simulink model "Pendulum"  (R2020b)
settings: Solver=VariableStepAuto  StartTime=0.0  StopTime=20  RelTol=1e-3
values from neighbouring files (symbols this model uses):
  A = [0, 0, 0; 0, 0 , 1; 0, 3*param.g/4/param.l, 0]    [InitPendulumController.m]
  B = [1; 0; 3/4/param.l]    [InitPendulumController.m]
  C = [1, 0, 0; 0, 0, 1]    [InitPendulumController.m]
  L_nom = place(A',C',p_nom)'    [InitPendulumController.m]
  ricatti_controller = lqr(A,B,Q,S)    [InitPendulumController.m]
  T_end = 1.5    [InitPendulumController.m]
  x = double(x1(order))    [InitPendulumController.m]    (also in Visualization.m = -L*sin(phi(idx)))
undefined symbols (not defined in the file or in its folder): ddwandler, DiscIntNeverNeededParam, param, veloctiycontroller
libraries: simulink x5
settings Model: Creator=Rolle  LastModifiedBy=klaus
settings DataIOCC: ReturnWorkspaceOutputs=off
settings DebuggingCC: ArithmeticOperatorsInVariantConditions=warning
settings SFSimCC: SimUseLocalCustomCode=off  CustomCodeUndefinedFunction=UseInterfaceOnly
settings RTWCC: RTWUseLocalCustomCode=off
settings CodeAppCC: StateflowObjectComments=on

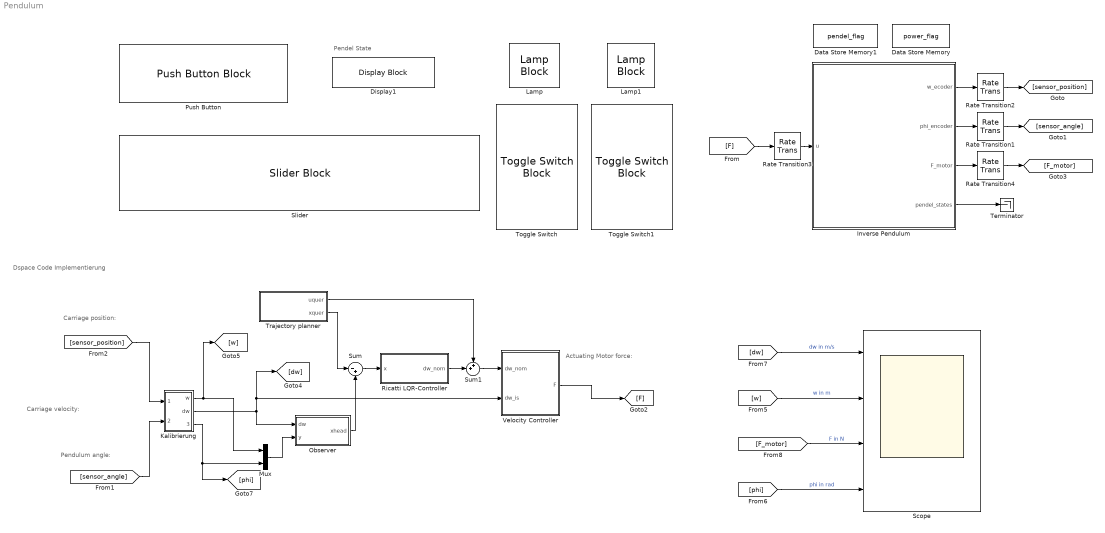
== system Pendulum ==
  note: Carriage position:
  note: Pendel State
  note: Dspace Code Implementierung
  note: Carriage velocity:
  note: Pendulum angle:
  note: Actuating Motor force:
  Data Store Memory : DataStoreMemory  DataStoreName=power_flag  ReadBeforeWriteMsg=warning  WriteAfterWriteMsg=warning  WriteAfterReadMsg=warning  ShowAdditionalParam=off  OutDataTypeStr=boolean
  Data Store Memory1 : DataStoreMemory  DataStoreName=pendel_flag  ReadBeforeWriteMsg=warning  WriteAfterWriteMsg=warning  WriteAfterReadMsg=warning  ShowAdditionalParam=off  OutDataTypeStr=boolean
  Display1 : DisplayBlock  LabelPosition=Hide
  Inverse Pendulum : Subsystem  mask(Inverses Pendel){wagen_flg=off}
      mask prompts: wagen_flg "Aufbau ohne Pendelaufsatz"
      mask help:
      | Schema des stehen Pendels: siehe Skript Abbildung 2.1
      |
      | Kraft ... F
      | Wagenbosition ... w
      | Pendelwinkel ... phi
  Kalibrierung : Subsystem
  Lamp : LampBlock  LabelPosition=Hide
  Lamp1 : LampBlock  LabelPosition=Hide
  Mux : Mux  Inputs=2
  Observer : Subsystem
  Push Button : PushButtonBlock  ButtonText=Disturbe
  Rate Transition1 : RateTransition  OutPortSampleTime=ctr.Ts2
  Rate Transition2 : RateTransition  OutPortSampleTime=ctr.Ts2
  Rate Transition3 : RateTransition
  Rate Transition4 : RateTransition  OutPortSampleTime=ctr.Ts2
  Ricatti LQR-Controller : Subsystem
  Scope : Scope  NumInputPorts=4
  Slider : SliderBlock  ScaleMin=-10  ScaleMax=10
  Sum : Sum  Inputs=|-+
  Sum1 : Sum  Inputs=++|
  Terminator : Terminator
  Toggle Switch : ToggleSwitchBlock
      settings: Values={{'Off', 'On'}, [0 1]}
  Toggle Switch1 : ToggleSwitchBlock
      settings: Values={{'Off', 'On'}, [0 1]}
  Trajectory planner : Subsystem
  Velocity Controller : Subsystem
  wires:
  Inverse Pendulum/2(phi_encoder) -> Rate Transition1/1
  Rate Transition3/1 -> Inverse Pendulum/1(u)
  Inverse Pendulum/1(w_ecoder) -> Rate Transition2/1
  Rate Transition2/1 -> [sensor_position]
  Rate Transition1/1 -> [sensor_angle]
  [F] -> Rate Transition3/1
  Inverse Pendulum/3(F_motor) -> Rate Transition4/1
  Rate Transition4/1 -> [F_motor]
  Inverse Pendulum/4(pendel_states) -> Terminator/1
  Velocity Controller/1(F) -> [F]
  [dw] -> Scope/1  "dw in m/s"
  [w] -> Scope/2  "w in m"
  [F_motor] -> Scope/3  "F in N"
  [phi] -> Scope/4  "phi in rad"
  [sensor_position] -> Kalibrierung/1(In1)
  [sensor_angle] -> Kalibrierung/2(In2)
  Kalibrierung/1(w) -> Mux/1, [w]
  Kalibrierung/3(phi) -> Mux/2, [phi]
  Mux/1 -> Observer/2(y)
  Kalibrierung/2(dw) -> Observer/1(dw), [dw], Velocity Controller/2(dw_is)
  Trajectory planner/2(xquer) -> Sum/1
  Sum1/1 -> Velocity Controller/1(dw_nom)
  Trajectory planner/1(uquer) -> Sum1/1
  Sum/1 -> Ricatti LQR-Controller/1(x)
  Observer/1(xhead) -> Sum/2
  Ricatti LQR-Controller/1(dw_nom) -> Sum1/2

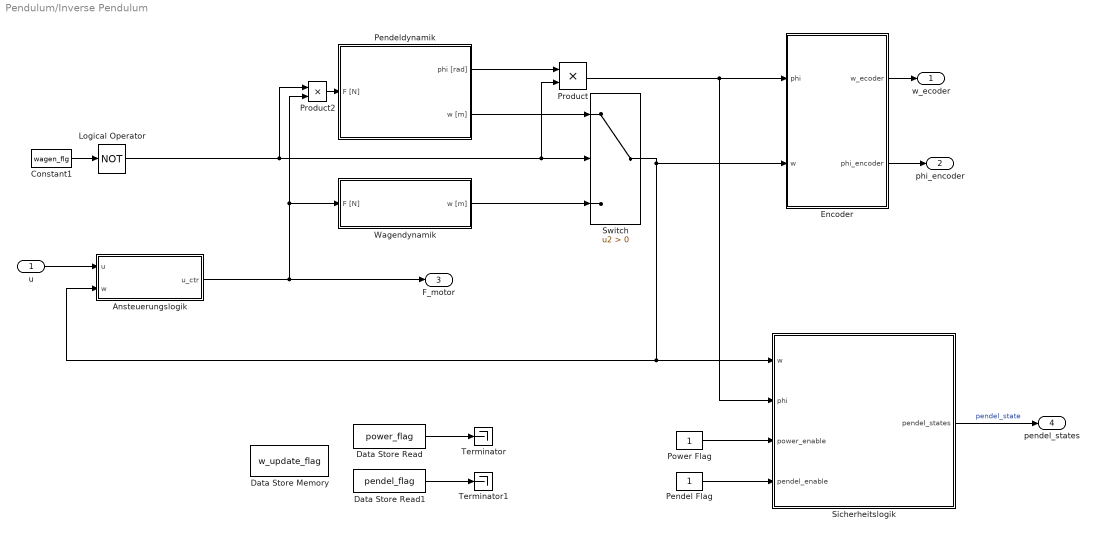
== system Pendulum/Inverse Pendulum ==
  u : Inport  OutDataTypeStr=double
  Ansteuerungslogik : Subsystem
  Constant1 : Constant  Value=wagen_flg
  Data Store Memory : DataStoreMemory  DataStoreName=w_update_flag  ReadBeforeWriteMsg=warning  WriteAfterWriteMsg=warning  WriteAfterReadMsg=warning  ShowAdditionalParam=off  OutDataTypeStr=boolean
  Data Store Read : DataStoreRead  DataStoreName=power_flag
  Data Store Read1 : DataStoreRead  DataStoreName=pendel_flag
  Encoder : Subsystem
  Logical Operator : Logic  Operator=NOT  AllPortsSameDT=off  OutDataTypeStr=boolean
  Pendel Flag : Constant  OutDataTypeStr=boolean
  Pendeldynamik : Subsystem
  "Power Flag " : Constant  OutDataTypeStr=boolean
  Product : Product
  Product2 : Product
  Sicherheitslogik : Subsystem
  Switch : Switch  Criteria=u2 > Threshold
  Terminator : Terminator
  Terminator1 : Terminator
  Wagendynamik : Subsystem
  w_ecoder : Outport  VectorParamsAs1DForOutWhenUnconnected=off
  phi_encoder : Outport  Port=2  VectorParamsAs1DForOutWhenUnconnected=off
  F_motor : Outport  Port=3  VectorParamsAs1DForOutWhenUnconnected=off
  pendel_states : Outport  Port=4  VectorParamsAs1DForOutWhenUnconnected=off
  wires:
  Constant1/1 -> Logical Operator/1
  Wagendynamik/1(w [m]) -> Switch/3
  Pendeldynamik/1(phi [rad]) -> Product/1
  Pendeldynamik/2(w [m]) -> Switch/1
  Logical Operator/1 -> Product2/1, Product/2, Switch/2
  Data Store Read/1 -> Terminator/1
  Data Store Read1/1 -> Terminator1/1
  Product/1 -> Sicherheitslogik/2(phi), Encoder/1(phi)
  Switch/1 -> Ansteuerungslogik/2(w), Sicherheitslogik/1(w), Encoder/2(w)
  Encoder/1(w_ecoder) -> w_ecoder/1
  Encoder/2(phi_encoder) -> phi_encoder/1
  Product2/1 -> Pendeldynamik/1(F [N])
  Ansteuerungslogik/1(u_ctr) -> Product2/2, Wagendynamik/1(F [N]), F_motor/1
  u/1 -> Ansteuerungslogik/1(u)
  "Power Flag "/1 -> Sicherheitslogik/3(power_enable)
  Pendel Flag/1 -> Sicherheitslogik/4(pendel_enable)
  Sicherheitslogik/1(pendel_states) -> pendel_states/1  "pendel_state"

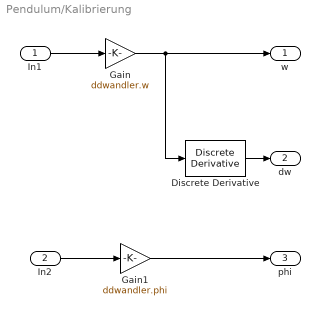
== system Pendulum/Kalibrierung ==
  In1 : Inport
  In2 : Inport  Port=2
  Discrete Derivative : simulink/Discrete/Discrete Derivative  gainval=1.0  ICPrevScaledInput=0.0  OutMin=[]  OutMax=[]  OutDataType=fixdt(1, 16)  OutScaling=2^-10  DoSatur=off
  Gain : Gain  Gain=ddwandler.w
  Gain1 : Gain  Gain=ddwandler.phi
  w : Outport
  dw : Outport  Port=2
  phi : Outport  Port=3
  wires:
  In2/1 -> Gain1/1
  In1/1 -> Gain/1
  Gain1/1 -> phi/1
  Gain/1 -> Discrete Derivative/1, w/1
  Discrete Derivative/1 -> dw/1

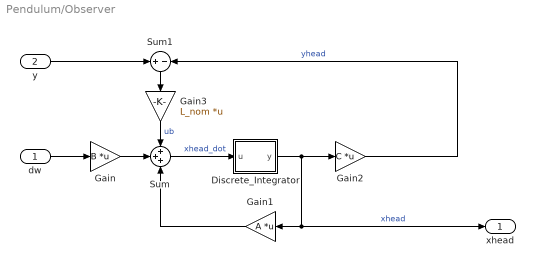
== system Pendulum/Observer ==
  dw : Inport
  y : Inport  Port=2
  Discrete_Integrator : Subsystem
  Gain : Gain  Gain=B  Multiplication=Matrix(K*u)
  Gain1 : Gain  Gain=A  Multiplication=Matrix(K*u)
  Gain2 : Gain  Gain=C  Multiplication=Matrix(K*u)
  Gain3 : Gain  Gain=L_nom  Multiplication=Matrix(K*u)
  Sum : Sum  Inputs=+++
  Sum1 : Sum  Inputs=+|-
  xhead : Outport
  wires:
  dw/1 -> Gain/1
  Discrete_Integrator/1(y) -> Gain2/1, xhead/1, Gain1/1  "xhead"
  Sum/1 -> Discrete_Integrator/1(u)  "xhead_dot"
  Gain/1 -> Sum/2
  Gain1/1 -> Sum/3
  Gain2/1 -> Sum1/2  "yhead"
  y/1 -> Sum1/1
  Sum1/1 -> Gain3/1
  Gain3/1 -> Sum/1  "ub"

== system Pendulum/Ricatti LQR-Controller ==
  x : Inport
  Gain1 : Gain  Gain=-1
  Ricatti LQR controller : Gain  Gain=ricatti_controller  Multiplication=Matrix(K*u) (u vector)
  dw_nom : Outport
  wires:
  Ricatti LQR controller/1 -> Gain1/1
  Gain1/1 -> dw_nom/1
  x/1 -> Ricatti LQR controller/1

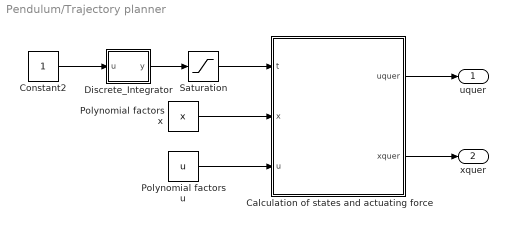
== system Pendulum/Trajectory planner ==
  Calculation of states and actuating force : MATLAB Function  TreatAsAtomicUnit=on
  Constant2 : Constant
  Discrete_Integrator : Subsystem
  Polynomial factors u : Constant  Value=u
  Polynomial factors x : Constant  Value=x
  Saturation : Saturate  UpperLimit=T_end  LowerLimit=0
  uquer : Outport
  xquer : Outport  Port=2
  wires:
  Discrete_Integrator/1(y) -> Saturation/1
  Calculation of states and actuating force/1(uquer) -> uquer/1
  Calculation of states and actuating force/2(xquer) -> xquer/1
  Polynomial factors x/1 -> Calculation of states and actuating force/2(x)
  Polynomial factors u/1 -> Calculation of states and actuating force/3(u)
  Saturation/1 -> Calculation of states and actuating force/1(t)
  Constant2/1 -> Discrete_Integrator/1(u)

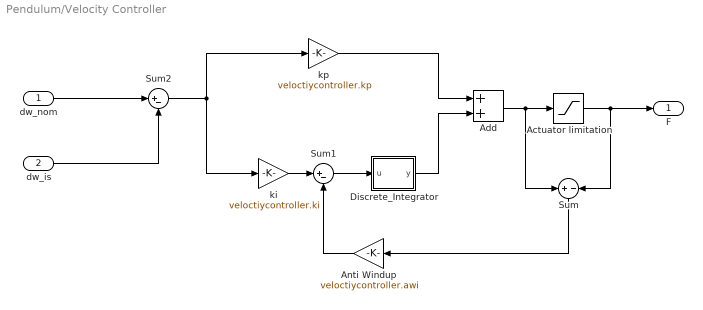
== system Pendulum/Velocity Controller ==
  dw_nom : Inport
  dw_is : Inport  Port=2
  Actuator limitation : Saturate  UpperLimit=95  LowerLimit=-95
  Add : Sum
  Anti Windup : Gain  Gain=veloctiycontroller.awi
  Discrete_Integrator : Subsystem
  Sum : Sum  Inputs=+|-
  Sum1 : Sum  Inputs=|+-
  Sum2 : Sum  Inputs=|+-
  ki : Gain  Gain=veloctiycontroller.ki
  kp : Gain  Gain=veloctiycontroller.kp
  F : Outport
  wires:
  Discrete_Integrator/1(y) -> Add/2
  Sum2/1 -> ki/1, kp/1
  kp/1 -> Add/1
  Actuator limitation/1 -> Sum/2, F/1
  Add/1 -> Sum/1, Actuator limitation/1
  Sum/1 -> Anti Windup/1
  ki/1 -> Sum1/1
  Anti Windup/1 -> Sum1/2
  Sum1/1 -> Discrete_Integrator/1(u)
  dw_is/1 -> Sum2/2
  dw_nom/1 -> Sum2/1

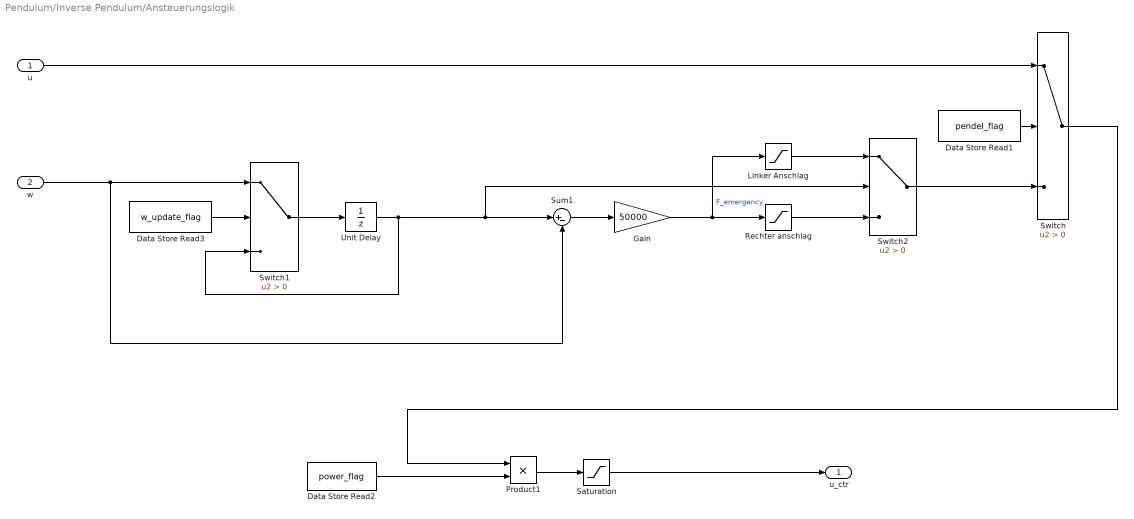
== system Pendulum/Inverse Pendulum/Ansteuerungslogik ==
  u : Inport
  w : Inport  Port=2
  Data Store Read1 : DataStoreRead  DataStoreName=pendel_flag
  Data Store Read2 : DataStoreRead  DataStoreName=power_flag
  Data Store Read3 : DataStoreRead  DataStoreName=w_update_flag
  Gain : Gain  Gain=50000
  Linker Anschlag : Saturate  UpperLimit=10  LowerLimit=-inf
  Product1 : Product
  Rechter anschlag : Saturate  UpperLimit=inf  LowerLimit=-10
  Saturation : Saturate  UpperLimit=99.83  LowerLimit=-99.83
  Sum1 : Sum  Inputs=|+-
  Switch : Switch  Criteria=u2 > Threshold
  Switch1 : Switch  Criteria=u2 > Threshold
  Switch2 : Switch  Criteria=u2 > Threshold
  Unit Delay : UnitDelay  SampleTime=-1  HasFrameUpgradeWarning=on
  u_ctr : Outport  VectorParamsAs1DForOutWhenUnconnected=off
  wires:
  Product1/1 -> Saturation/1
  Data Store Read2/1 -> Product1/2
  Sum1/1 -> Gain/1
  Linker Anschlag/1 -> Switch2/1
  Gain/1 -> Linker Anschlag/1, Rechter anschlag/1  "F_emergency"
  Switch1/1 -> Unit Delay/1
  Switch2/1 -> Switch/3
  Data Store Read3/1 -> Switch1/2
  Unit Delay/1 -> Switch2/2, Sum1/1, Switch1/3
  Rechter anschlag/1 -> Switch2/3
  w/1 -> Sum1/2, Switch1/1
  u/1 -> Switch/1
  Data Store Read1/1 -> Switch/2
  Switch/1 -> Product1/1
  Saturation/1 -> u_ctr/1

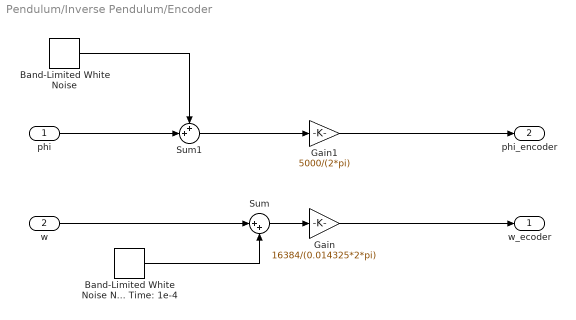
== system Pendulum/Inverse Pendulum/Encoder ==
  phi : Inport
  w : Inport  Port=2
  Band-Limited White Noise : simulink/Sources/Band-Limited White Noise  Cov=1e-25  Ts=1e-4  seed=[23341]
  "Band-Limited White Noise Noise Power: 1e-15 -> reuslting in [-1, 1]e-5  deviation Sample Time: 1e-4" : simulink/Sources/Band-Limited White Noise  Cov=1e-15  Ts=1e-4  seed=[23341]
  Gain : Gain  Gain=16384/(0.014325*2*pi)
  Gain1 : Gain  Gain=5000/(2*pi)
  Sum : Sum  Inputs=|++
  Sum1 : Sum  Inputs=++|
  w_ecoder : Outport  VectorParamsAs1DForOutWhenUnconnected=off
  phi_encoder : Outport  Port=2  VectorParamsAs1DForOutWhenUnconnected=off
  wires:
  w/1 -> Sum/1
  Sum1/1 -> Gain1/1
  "Band-Limited White Noise Noise Power: 1e-15 -> reuslting in [-1, 1]e-5  deviation Sample Time: 1e-4"/1 -> Sum/2
  Sum/1 -> Gain/1
  Gain1/1 -> phi_encoder/1
  Gain/1 -> w_ecoder/1
  Band-Limited White Noise/1 -> Sum1/1
  phi/1 -> Sum1/2

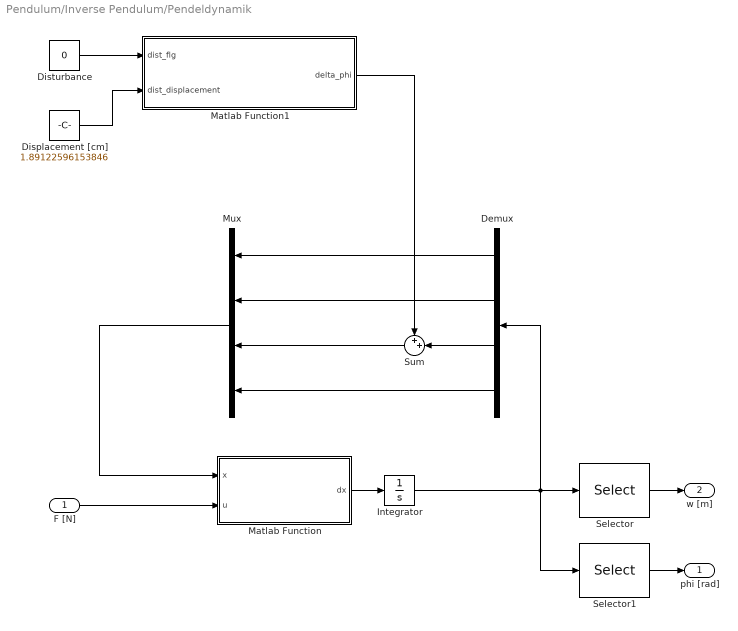
== system Pendulum/Inverse Pendulum/Pendeldynamik ==
  F [N] : Inport
  Demux : Demux
  Displacement [cm] : Constant  Value=1.89122596153846
  Disturbance : Constant  Value=0  OutDataTypeStr=boolean
  Integrator : Integrator  InitialCondition=[0 0 0 0]'
  Matlab Function : MATLAB Function  TreatAsAtomicUnit=on
  Matlab Function1 : MATLAB Function  TreatAsAtomicUnit=on
  Mux : Mux
  Selector : Selector  InputPortWidth=4  IndexOptions=Index vector (dialog)  Indices=[1]  OutputSizes=1
  Selector1 : Selector  InputPortWidth=4  IndexOptions=Index vector (dialog)  Indices=[3]  OutputSizes=1
  Sum : Sum  Inputs=++|
  phi [rad] : Outport  VectorParamsAs1DForOutWhenUnconnected=off
  w [m] : Outport  Port=2  VectorParamsAs1DForOutWhenUnconnected=off
  wires:
  Matlab Function/1(dx) -> Integrator/1
  Integrator/1 -> Demux/1, Selector1/1, Selector/1
  F [N]/1 -> Matlab Function/2(u)
  Selector/1 -> w [m]/1
  Selector1/1 -> phi [rad]/1
  Demux/4 -> Mux/4
  Demux/1 -> Mux/1
  Demux/2 -> Mux/2
  Demux/3 -> Sum/2
  Sum/1 -> Mux/3
  Mux/1 -> Matlab Function/1(x)
  Disturbance/1 -> Matlab Function1/1(dist_flg)
  Matlab Function1/1(delta_phi) -> Sum/1
  Displacement [cm]/1 -> Matlab Function1/2(dist_displacement)

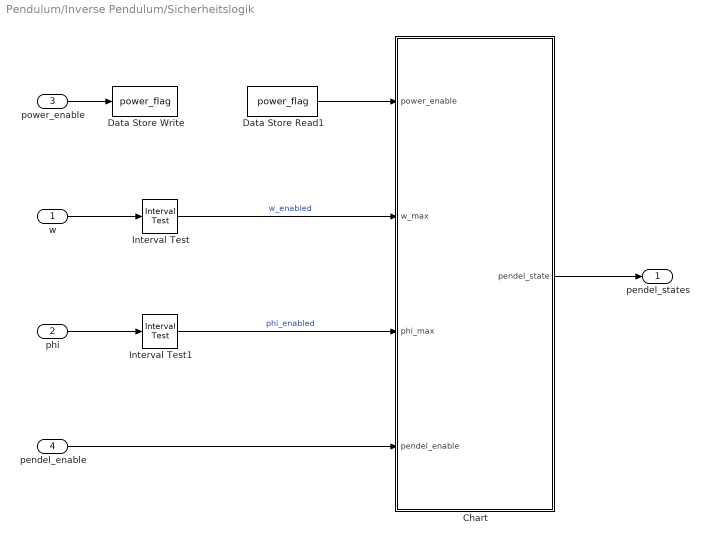
== system Pendulum/Inverse Pendulum/Sicherheitslogik ==
  w : Inport
  phi : Inport  Port=2
  power_enable : Inport  Port=3
  pendel_enable : Inport  Port=4
  Chart : Stateflow chart  TreatAsAtomicUnit=on
  Data Store Read1 : DataStoreRead  DataStoreName=power_flag
  Data Store Write : DataStoreWrite  DataStoreName=power_flag
  Interval Test : simulink/Logic and Bit Operations/Interval Test  IntervalClosedRight=on  uplimit=0.4  IntervalClosedLeft=on  lowlimit=-0.4  OutDataTypeStr=boolean
  Interval Test1 : simulink/Logic and Bit Operations/Interval Test  IntervalClosedRight=on  uplimit=20*pi/180  IntervalClosedLeft=on  lowlimit=-20*pi/180  OutDataTypeStr=boolean
  pendel_states : Outport  VectorParamsAs1DForOutWhenUnconnected=off
  wires:
  power_enable/1 -> Data Store Write/1
  Interval Test/1 -> Chart/2(w_max)  "w_enabled"
  w/1 -> Interval Test/1
  Interval Test1/1 -> Chart/3(phi_max)  "phi_enabled"
  pendel_enable/1 -> Chart/4(pendel_enable)
  Data Store Read1/1 -> Chart/1(power_enable)
  Chart/1(pendel_state) -> pendel_states/1
  phi/1 -> Interval Test1/1

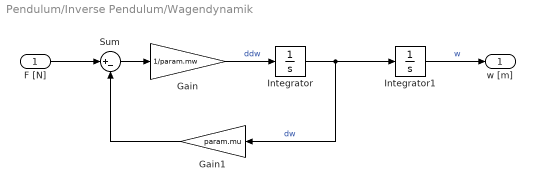
== system Pendulum/Inverse Pendulum/Wagendynamik ==
  F [N] : Inport
  Gain : Gain  Gain=1/param.mw
  Gain1 : Gain  Gain=param.mu
  Integrator : Integrator
  Integrator1 : Integrator
  Sum : Sum  Inputs=|+-
  w [m] : Outport  VectorParamsAs1DForOutWhenUnconnected=off
  wires:
  Sum/1 -> Gain/1
  Integrator/1 -> Gain1/1, Integrator1/1  "dw"
  Gain/1 -> Integrator/1  "ddw"
  Gain1/1 -> Sum/2
  F [N]/1 -> Sum/1
  Integrator1/1 -> w [m]/1  "w"

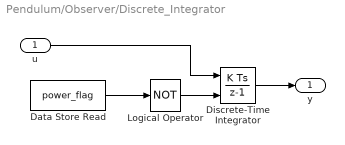
== system Pendulum/Observer/Discrete_Integrator ==
  u : Inport
  Data Store Read : DataStoreRead  DataStoreName=power_flag
  Discrete-Time Integrator : DiscreteIntegrator  ExternalReset=level  SampleTime=-1  ICPrevOutput=DiscIntNeverNeededParam  ICPrevScaledInput=DiscIntNeverNeededParam
  Logical Operator : Logic  Operator=NOT  AllPortsSameDT=off  OutDataTypeStr=boolean
  y : Outport  VectorParamsAs1DForOutWhenUnconnected=off
  wires:
  Logical Operator/1 -> Discrete-Time Integrator/2
  Data Store Read/1 -> Logical Operator/1
  u/1 -> Discrete-Time Integrator/1
  Discrete-Time Integrator/1 -> y/1

== system Pendulum/Trajectory planner/Discrete_Integrator ==
  u : Inport
  Data Store Read : DataStoreRead  DataStoreName=power_flag
  Discrete-Time Integrator : DiscreteIntegrator  ExternalReset=level  SampleTime=-1  ICPrevOutput=DiscIntNeverNeededParam  ICPrevScaledInput=DiscIntNeverNeededParam
  Logical Operator : Logic  Operator=NOT  AllPortsSameDT=off  OutDataTypeStr=boolean
  y : Outport  VectorParamsAs1DForOutWhenUnconnected=off
  wires:
  Logical Operator/1 -> Discrete-Time Integrator/2
  Data Store Read/1 -> Logical Operator/1
  u/1 -> Discrete-Time Integrator/1
  Discrete-Time Integrator/1 -> y/1

== system Pendulum/Velocity Controller/Discrete_Integrator ==
  u : Inport
  Data Store Read : DataStoreRead  DataStoreName=power_flag
  Discrete-Time Integrator : DiscreteIntegrator  ExternalReset=level  SampleTime=-1  ICPrevOutput=DiscIntNeverNeededParam  ICPrevScaledInput=DiscIntNeverNeededParam
  Logical Operator : Logic  Operator=NOT  AllPortsSameDT=off  OutDataTypeStr=boolean
  y : Outport  VectorParamsAs1DForOutWhenUnconnected=off
  wires:
  Logical Operator/1 -> Discrete-Time Integrator/2
  Data Store Read/1 -> Logical Operator/1
  u/1 -> Discrete-Time Integrator/1
  Discrete-Time Integrator/1 -> y/1

== matlab function Pendulum/Inverse Pendulum/Pendeldynamik/Matlab Function1 ==
  data: dist_flg input size=1; dist_displacement input size=1; delta_phi output size=1; param parameter
function delta_phi = fcn(dist_flg,dist_displacement,param)

delta_phi = dist_flg*asin(dist_displacement/100/(param.l*2));

== matlab function Pendulum/Inverse Pendulum/Pendeldynamik/Matlab Function ==
  data: x input double size=4; u input double size=1; dx output double size=4; param parameter
function dx = fcn(x,u,param)
%State #####
% x1 = w    ... position
% x2 = dw   ... velocity
% x3 = phi  ... pendulum angle
% x4 = dphi ... pendulum speed

%Input #####
% u = F  ... carriage force

Fg = u - param.mu*x(2); % Driving force
sphi = sin(x(3));  
cphi = cos(x(3));

%Parameter:
mpl = param.mp*param.l;
M = param.mc + param.mp;
J  = 4/3*mpl*param.l; 
MM  = M - (mpl*cphi)^2/J;
JJ = J -(mpl*cphi)^2/M;

%Tmp State:
mpldphisphi =  mpl*x(4)^2*sphi;
%System equation:
ddw   = (Fg + (mpl)^2*param.g/(2*J)*sin(2*x(3)) - mpldphisphi)/MM;
ddphi = (mpl*param.g*sphi  + mpl/M*cphi*(Fg - mpldphisphi))/JJ; 

dx = [x(2) ddw x(4) ddphi]';

== stateflow chart Pendulum/Inverse Pendulum/Sicherheitslogik/Chart ==
  state start/
    entry:
    pendel_flag=false;
    pendel_state=0;
    w_update_flag=true;
  state on/
    entry:
    pendel_flag=true;
    pendel_state=1;
    w_update_flag=true;
  state intermediate_start/
    % Verhindert ein
    % Springen des
    % Wagens wen etwas
    % nicht stimmt
  state emergency_off_power/
    % Power Fehler
    entry:
    pendel_flag=false;
    pendel_state=2;
    w_update_flag=true;
  state emergency_off_w_position/
    % Postionsfehler
    entry:
    pendel_flag=false;
    pendel_state=3;
    w_update_flag=false;
  state emergency_off_p_angle/
    % Winkelfehler
    entry:
    pendel_flag=false;
    pendel_state=4;
    w_update_flag=true;
  on -> start [order 4] : [pendel_enable~=1]
  start -> intermediate_start : [pendel_enable==1]
  intermediate_start -> on [order 4] : [pendel_enable==1]
  (default) -> start
  intermediate_start -> emergency_off_power [order 1] : [power_enable~=1]
  intermediate_start -> emergency_off_w_position [order 2] : [w_max~=1]
  intermediate_start -> emergency_off_p_angle [order 3] : [phi_max~=1]
  emergency_off_p_angle -> start [order 3] : [pendel_enable~=1]
  emergency_off_w_position -> start [order 2] : [pendel_enable~=1]
  emergency_off_power -> start : [pendel_enable~=1]
  on -> emergency_off_power [order 3] : [power_enable~=1]
  on -> emergency_off_w_position [order 1] : [w_max~=1]
  on -> emergency_off_p_angle [order 2] : [phi_max~=1]
  emergency_off_w_position -> emergency_off_power [order 1] : [power_enable~=1]
  emergency_off_p_angle -> emergency_off_power [order 2] : [power_enable~=1]
  emergency_off_p_angle -> emergency_off_w_position [order 1] : [w_max~=1]
  data: power_enable input; w_max input; phi_max input; pendel_enable input; pendel_flag data_store_memory; pendel_state output; w_update_flag data_store_memory

== matlab function Pendulum/Trajectory planner/Calculation of states and actuating force ==
  data: t input; uquer output; xquer output; x input; u input
function [uquer, xquer] = fcn(t, x, u)
  xquer = [x(1)*t^7+x(2)*t^6+x(3)*t^5+x(4)*t^4+x(5)*t^3+x(6)*t^2;...
  x(7)*t^6+x(8)*t^5+x(9)*t^4+x(10)*t^3;...
  x(11)*t^5+x(12)*t^4+x(13)*t^3+x(14)*t^2];
  uquer = u(1)*t^6 +u(2)*t^5+u(3)*t^4+u(4)*t^3+u(5)*t^2+u(6)*t;
end
